simulink model "iface"  (R2018b)
settings: Solver=FixedStepDiscrete  StartTime=0.0  StopTime=10.0  RelTol=1e-3
settings Model: Creator=matlab  LastModifiedBy=matlab

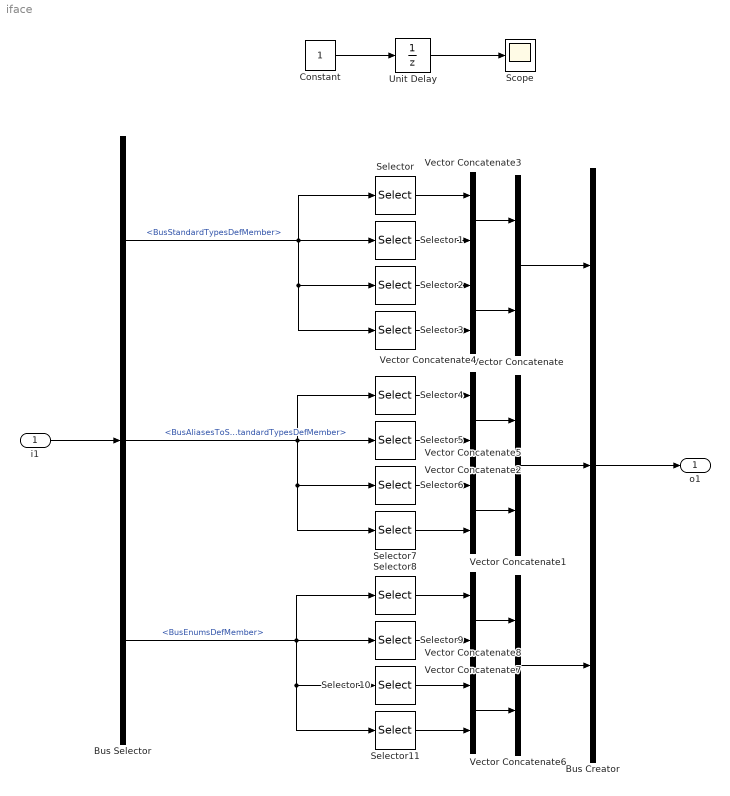
== system iface ==
  i1 : Inport  OutDataTypeStr=Bus: BusDef  BusOutputAsStruct=on
  Bus Creator : BusCreator  Inputs=3  OutDataTypeStr=Bus: BusDef  NonVirtualBus=on
      settings: InheritFromInputs=off
  Bus Selector : BusSelector  OutputSignals=BusStandardTypesDefMember,BusAliasesToStandardTypesDefMember,BusEnumsDefMember
  Constant : Constant
  Scope : Scope
  Selector : Selector  NumberOfDimensions=2  InputPortWidth=2  IndexOptions=Index vector (dialog),Index vector (dialog)  Indices=1,1  OutputSizes=1,1
  Selector1 : Selector  NumberOfDimensions=2  InputPortWidth=2  IndexOptions=Index vector (dialog),Index vector (dialog)  Indices=1,2  OutputSizes=1,1
  Selector10 : Selector  NumberOfDimensions=2  InputPortWidth=2  IndexOptions=Index vector (dialog),Index vector (dialog)  Indices=2,1  OutputSizes=1,1
  Selector11 : Selector  NumberOfDimensions=2  InputPortWidth=2  IndexOptions=Index vector (dialog),Index vector (dialog)  Indices=2,2  OutputSizes=1,1
  Selector2 : Selector  NumberOfDimensions=2  InputPortWidth=2  IndexOptions=Index vector (dialog),Index vector (dialog)  Indices=2,1  OutputSizes=1,1
  Selector3 : Selector  NumberOfDimensions=2  InputPortWidth=2  IndexOptions=Index vector (dialog),Index vector (dialog)  Indices=2,2  OutputSizes=1,1
  Selector4 : Selector  NumberOfDimensions=2  InputPortWidth=2  IndexOptions=Index vector (dialog),Index vector (dialog)  Indices=1,1  OutputSizes=1,1
  Selector5 : Selector  NumberOfDimensions=2  InputPortWidth=2  IndexOptions=Index vector (dialog),Index vector (dialog)  Indices=1,2  OutputSizes=1,1
  Selector6 : Selector  NumberOfDimensions=2  InputPortWidth=2  IndexOptions=Index vector (dialog),Index vector (dialog)  Indices=2,1  OutputSizes=1,1
  Selector7 : Selector  NumberOfDimensions=2  InputPortWidth=2  IndexOptions=Index vector (dialog),Index vector (dialog)  Indices=2,2  OutputSizes=1,1
  Selector8 : Selector  NumberOfDimensions=2  InputPortWidth=2  IndexOptions=Index vector (dialog),Index vector (dialog)  Indices=1,1  OutputSizes=1,1
  Selector9 : Selector  NumberOfDimensions=2  InputPortWidth=2  IndexOptions=Index vector (dialog),Index vector (dialog)  Indices=1,2  OutputSizes=1,1
  Unit Delay : UnitDelay  SampleTime=-1
  Vector Concatenate : Concatenate  Mode=Multidimensional array  ConcatenateDimension=2
  Vector Concatenate1 : Concatenate  Mode=Multidimensional array  ConcatenateDimension=2
  Vector Concatenate{2..5,7..8} (6 alike) : Concatenate  ConcatenateDimension=2
  Vector Concatenate6 : Concatenate  Mode=Multidimensional array  ConcatenateDimension=2
  o1 : Outport  OutDataTypeStr=Bus: BusDef
  wires:
  Unit Delay/1 -> Scope/1
  Constant/1 -> Unit Delay/1
  i1/1 -> Bus Selector/1
  Bus Selector/3 -> Selector9/1, Selector8/1, Selector11/1, Selector10/1  "<BusEnumsDefMember>"
  Bus Selector/2 -> Selector7/1, Selector6/1, Selector4/1, Selector5/1  "<BusAliasesToStandardTypesDefMember>"
  Bus Selector/1 -> Selector3/1, Selector2/1, Selector1/1, Selector/1  "<BusStandardTypesDefMember>"
  Vector Concatenate/1 -> Bus Creator/1
  Bus Creator/1 -> o1/1
  Selector/1 -> Vector Concatenate3/1
  Selector1/1 -> Vector Concatenate3/2
  Vector Concatenate3/1 -> Vector Concatenate/1
  Selector2/1 -> Vector Concatenate4/1
  Selector3/1 -> Vector Concatenate4/2
  Vector Concatenate4/1 -> Vector Concatenate/2
  Selector7/1 -> Vector Concatenate5/2
  Selector6/1 -> Vector Concatenate5/1
  Vector Concatenate2/1 -> Vector Concatenate1/1
  Selector5/1 -> Vector Concatenate2/2
  Selector4/1 -> Vector Concatenate2/1
  Vector Concatenate5/1 -> Vector Concatenate1/2
  Vector Concatenate1/1 -> Bus Creator/2
  Selector11/1 -> Vector Concatenate8/2
  Selector10/1 -> Vector Concatenate8/1
  Vector Concatenate7/1 -> Vector Concatenate6/1
  Selector9/1 -> Vector Concatenate7/2
  Selector8/1 -> Vector Concatenate7/1
  Vector Concatenate8/1 -> Vector Concatenate6/2
  Vector Concatenate6/1 -> Bus Creator/3
